simulink model "filtros_fir"  (R2014a)
settings: Solver=ode45  StartTime=0.0  StopTime=10.0  RelTol=1e-3
libraries: MCHP_Blockset x2
settings Model: Creator=Wels  LastModifiedBy=Wels

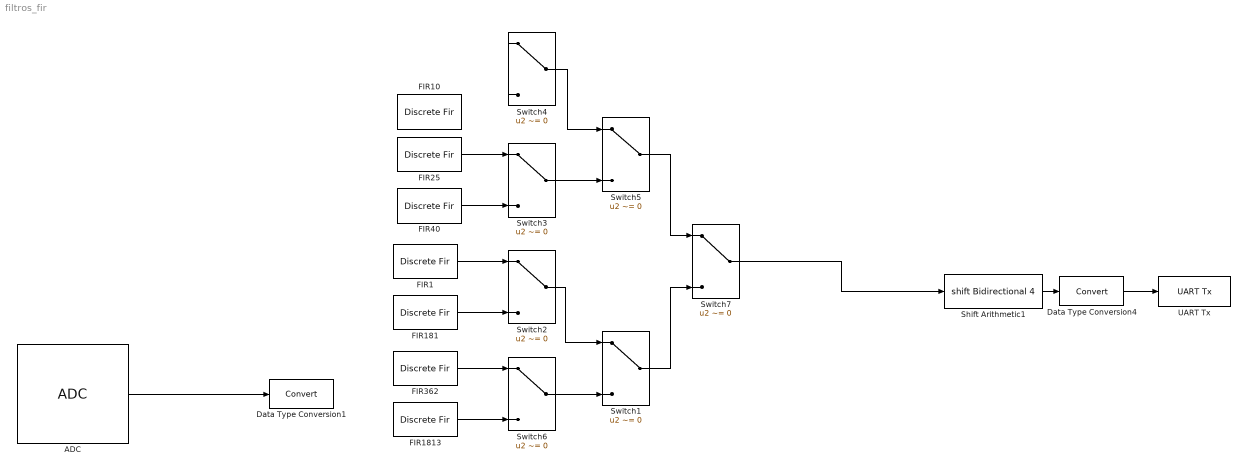
== system filtros_fir ==
  ADC : MCHP_Blockset/Analog IO/ADC  Priority=5  ADC_REF=1  Mode=12 bits  FORM=0000 dddd dddd dddd ==> Unsigned integer  ADC_R="< 5    kOhm"  nSAMPLECHANNELS=CH0 only  nSAMPLECHANNELS_12bits=CH0 only  SIMULTANEOUS=Simultaneously on all Channels  ADxCSS=[0]  MUXA_CH0N=off  MUXA_CH123=Dynamic Options  MUXA_CH123_TXT=AN0 : AN1 : AN2  MUXB_CH0=AN1  MUXB_CH0N=on  MUXB_CH123=Dynamic Options  MUXB_CH123_TXT=AN0 : AN1 : AN2  SequenceRepeat=1  SequenceTiming=are done as fast as possible at end of previous time step  SSRC_SSRCG=Dynamic Options  SSRC_SSRCG_TXT=0  Update_BlockOutput=After all trig and conversion sequence  Trig_TimeStep=with each update of the ADC block output  ADC_DMA_CHANNEL=use DMA Channel 0  SampleTime=0.001  Info=Total Time for Sample & Conversion : 9.45e-06s including 0s (x 1) sample time.  MCHP_PORT={Analog Input 0}{AN0}15:2:A0;  MCHP_MASTERLINK=ADC_DSPIC33/Microchip Master  ADC_TIMING=[9.4499999999999993e-06]
  Data Type Conversion1 : DataTypeConversion
  Data Type Conversion4 : DataTypeConversion
  FIR1 : DiscreteFir  Tag=BlockMethodSubSystem  Coefficients=[-2.9323800933922057e-18 -0.0015228449366636073 -0.003018760535505417 -0.0043911540093978458 -0.0055466659235829602 -0.006401109439598384 -0.0068851121818910791 -0.0069491080760650491 -0.0065673515956200142 -0.0057406721770929675 -0.0044977500977790479 -0.002894773705028665 -0.0010134274197902613 0.0010427444668100105 0.0031534568919988934 0.0051880532674748276 0.0070128109723885373 0.0084988032998812423 0.0095298916645369987 0.010010398197200024 0.0098720098997901601 0.009079491954896806 0.0076348388043248989 0.0055795650340087688 0.0029949304160725048 -3.0714546289964412e-18 -0.003252444656358322 -0.0065820093502685917 -0.0097885587309644792 -0.012661504624490524 -0.014990073316292731 -0.016574048280221781 -0.017234444684547753 -0.016823560059853641 -0.015233863006149173 -0.012405228378154698 -0.0083301010511404264 -0.0030562676555698828 0.0033129682426820939 0.010621283060200347 0.01866444257636788 0.027197829873822289 0.035946071730047706 0.0446143319962145 0.052900750057141198 0.060509437929656872 0.06716341457002048 0.072616852612101865 0.076666041454452896 0.079158530052541462 0.080000000000000002 0.079158530052541462 0.076666041454452896 0.072616852612101865 0.06716341457002048 0.060509437929656872 0.052900750057141198 0.0446143319962145 0.035946071730047706 0.027197829873822289 0.01866444257636788 0.010621283060200347 0.0033129682426820939 -0.0030562676555698828 -0.0083301010511404264 -0.012405228378154698 -0.015233863006149173 -0.016823560059853641 -0.017234444684547753 -0.016574048280221781 -0.014990073316292731 -0.012661504624490524 -0.0097885587309644792 -0.0065820093502685917 -0.003252444656358322 -3.0714546289964412e-18 0.0029949304160725048 0.0055795650340087688 0.0076348388043248989 0.009079491954896806 0.0098720098997901601 0.010010398197200024 0.0095298916645369987 0.0084988032998812423 0.0070128109723885373 0.0051880532674748276 0.0031534568919988934 0.0010427444668100105 -0.0010134274197902613 -0.002894773705028665 -0.0044977500977790479 -0.0057406721770929675 -0.0065673515956200142 -0.0069491080760650491 -0.0068851121818910791 -0.006401109439598384 -0.0055466659235829602 -0.0043911540093978458 -0.003018760535505417 -0.0015228449366636073 -2.9323800933922057e-18]  InputProcessing=Columns as channels (frame based)
  FIR10 : DiscreteFir  Tag=BlockMethodSubSystem  Coefficients=[0.05693190881682296 0.064608222044922184 0.071056300974898803 0.075931585257515435 0.078968604608715479 0.080000000000000002 0.078968604608715479 0.075931585257515435 0.071056300974898803 0.064608222044922184 0.05693190881682296]  InputProcessing=Columns as channels (frame based)
  FIR181 : DiscreteFir  Tag=BlockMethodSubSystem  Coefficients=[-0.0022639883275030691 -0.0016133097538512582 -0.00084337344267178184 2.9443416248695584e-18 0.00086517641377111313 0.0016978131053387859 0.0024442123003697996 0.0030547195836404385 0.0034869560845998604 0.003708678283102423 0.0037000773326903952 0.0034553599178999222 0.0029834933057486866 0.0023080461643020054 0.0014661110869005709 0.00050635136262791396 -0.00051373005733820136 -0.0015311506685924538 -0.0024812459539193805 -0.0033016804917040386 -0.0039364294880122191 -0.0043394827542988946 -0.0044780334288872089 -0.0043349388843936772 -0.0039102801218845766 -0.0032218965099678034 -0.0023048322069548306 -0.0012096956199982533 3.0290297657205514e-18 0.0012513822618214151 0.0024664608508178859 0.0035668251972659718 0.0044785243876568756 0.0051368355744426308 0.0054906248202151566 0.0055060198236647657 0.0051691468796323733 0.0044877332357838159 0.0034914382478542848 0.00223084906371908 0.0007751549565775495 -0.00079140561269844506 -0.0023741542968877447 -0.0038733985661101879 -0.005190376874854942 -0.0062333851575417194 -0.0069237239799580944 -0.0072011036523168346 -0.0070281638123607104 -0.0063938039032713691 -0.0053150798729646688 -0.0038374974349784778 -0.0020336194772699002 3.0861621459651029e-18 0.0021474459298498633 0.0042794328011263498 0.0062603671781829252 0.0079561219027827548 0.0092421084067647388 0.010011201898530072 0.010181066581124654 0.0097004455811658952 0.0085540225930631104 0.00676552764947183 0.0043988448641004351 0.0015569812197178019 -0.0016211327142456927 -0.0049659227570060362 -0.0082843295155859021 -0.011368535968756527 -0.01400586195480538 -0.015989349523563991 -0.017128513034918618 -0.017259704669759533 -0.016255551437491036 -0.014032954062411557 -0.010559199993407797 -0.0058558293809127396 3.1149317064883305e-18 0.0068767805961167097 0.014592556181376771 0.022921323366296955 0.031601672190584421 0.040347287698284315 0.048858835554886501 0.05683667922089531 0.063993828108091844 0.070068498248876995 0.074835680459695922 0.078117155278273911 0.079789466969549874 0.079789466969549874 0.078117155278273911 0.074835680459695922 0.070068498248876995 0.063993828108091844 0.05683667922089531 0.048858835554886501 0.040347287698284315 0.031601672190584421 0.022921323366296955 0.014592556181376771 0.0068767805961167097 3.1149317064883305e-18 -0.0058558293809127396 -0.010559199993407797 -0.014032954062411557 -0.016255551437491036 -0.017259704669759533 -0.017128513034918618 -0.015989349523563991 -0.01400586195480538 -0.011368535968756527 -0.0082843295155859021 -0.0049659227570060362 -0.0016211327142456927 0.0015569812197178019 0.0043988448641004351 0.00676552764947183 0.0085540225930631104 0.0097004455811658952 0.010181066581124654 0.010011201898530072 0.0092421084067647388 0.0079561219027827548 0.0062603671781829252 0.0042794328011263498 0.0021474459298498633 3.0861621459651029e-18 -0.0020336194772699002 -0.0038374974349784778 -0.0053150798729646688 -0.0063938039032713691 -0.0070281638123607104 -0.0072011036523168346 -0.0069237239799580944 -0.0062333851575417194 -0.005190376874854942 -0.0038733985661101879 -0.0023741542968877447 -0.00079140561269844506 0.0007751549565775495 0.00223084906371908 0.0034914382478542848 0.0044877332357838159 0.0051691468796323733 0.0055060198236647657 0.0054906248202151566 0.0051368355744426308 0.0044785243876568756 0.0035668251972659718 0.0024664608508178859 0.0012513822618214151 3.0290297657205514e-18 -0.0012096956199982533 -0.0023048322069548306 -0.0032218965099678034 -0.0039102801218845766 -0.0043349388843936772 -0.0044780334288872089 -0.0043394827542988946 -0.0039364294880122191 -0.0033016804917040386 -0.0024812459539193805 -0.0015311506685924538 -0.00051373005733820136 0.00050635136262791396 0.0014661110869005709 0.0023080461643020054 0.0029834933057486866 0.0034553599178999222 0.0037000773326903952 0.003708678283102423 0.0034869560845998604 0.0030547195836404385 0.0024442123003697996 0.0016978131053387859 0.00086517641377111313 2.9443416248695584e-18 -0.00084337344267178184 -0.0016133097538512582 -0.0022639883275030691]  InputProcessing=Columns as channels (frame based)
  FIR1813 : DiscreteFir  Tag=BlockMethodSubSystem  Coefficients=[0.00032952911187119737 0.00032473517058408992 0.00029949947214209755 0.00025535873427201875 0.00019504278155501242 0.00012230579388882381 4.1692698517550693e-05 -4.1744761582324127e-05 -0.00012276454860099542 -0.00019626361161977597 -0.00025759924854245692 -0.00030288231409216285 -0.00032922376001048669 -0.00033491888265804487 -0.00031955753227915043 -0.00028405316575898459 -0.00023058871159179856 -0.00016248244320140519 -8.3982096279824835e-05 -6.6378809126254589e-19 8.4194265639719084e-05 0.00016330446084229693 0.00023234078908090157 0.00028693456551297903 0.00032361461065292786 0.00034002788653010461 0.00033509035547182875 0.00030905839515836395 0.00026351607613477046 0.00020127888834994712 0.00012621976019108465 4.3028116193721218e-05 -4.3083041127590029e-05 -0.00012670373238769583 -0.00020256682711292391 -0.00026587975187858034 -0.0003126271945743762 -0.00033982568954094315 -0.00034571394614225253 -0.00032986678380497633 -0.00029322531066992586 -0.00023804123246993393 -0.0001677385741200386 -8.6701299773445198e-05 1.7095769056652346e-18 8.6925318595543704e-05 0.00016860650087831315 0.00023989116296424423 0.00029626763732437309 0.00033415045389244166 0.00035110829718730557 0.00034601995103387403 0.00031914823459720516 0.0002721270659772768 0.00020786224138893871 0.00013035194690182514 4.4438084316086506e-05 -4.4496126492876797e-05 -0.00013086338682871302 -0.0002092232772418191 -0.00027462489353193199 -0.00032291958567181065 -0.00035102404877583029 -0.00035711708646546684 -0.00034075749539601774 -0.00030291544841017098 -0.0002459151748724359 -0.0001732923105356631 -8.9574665622856739e-05 4.2406091449575885e-18 8.9811607478043859e-05 0.00017421030583805502 0.00024787182406707563 0.00030613328248453022 0.00034528828751800633 0.0003628226390728592 0.00035757566579229744 0.00032981684192100972 0.00028123264099433977 0.00021482421448547933 0.00013472209444100291 4.5929355051342866e-05 -4.5990801287047665e-05 -0.0001352635294002786 -0.00021626507313371292 -0.00028387696388909773 -0.00033380938205546812 -0.00036287325745926619 -0.00036918385463395836 -0.00035228285218252104 -0.00031317101754854693 -0.00025424918107297564 -0.00017917097527751953 -9.2616364891862638e-05 6.9431773108757513e-18 9.2867437590043943e-05 0.00018014371864827212 0.00025632252324914645 0.00031658076277386844 0.00035708386391707981 0.00037522969629670582 0.00036981563229449645 0.00034111802080524176 0.0002908788368540374 0.00022220009372350599 0.00013935240789474931 4.7509524650286494e-05 -4.7574698191683825e-05 -0.0001399266862029288 -0.00022372835517093937 -0.00029368356651569014 -0.00034535275480525611 -0.00037543458956305632 -0.0003819768071617564 -0.0003645027548861563 -0.00032404545418710423 -0.00026308678495157249 -0.00018540535425814439 -9.5842367054886074e-05 -1.1357237884133027e-18 9.6108934286664861e-05 0.00018643812916845751 0.00026528808170405533 0.00032766563145260981 0.00036960006498509737 0.00038839577976460714 0.00038280543597178358 0.00035311248165536272 0.00030111760635609418 0.00023002970645582749 0.00014426795378438256 4.9187169506072944e-05 -4.9256436000125337e-05 -0.00014487829737313407 -0.00023165394499001139 -0.00030409847902950876 -0.00035761316967114259 -0.00038877728673591022 -0.00039556664557550373 -0.0003774849135906076 -0.00033559917005555645 -0.00027247721077334916 -0.00019203026271991702 -9.9270734439122545e-05 1.5660508920444814e-18 9.9554341743169492e-05 0.00019312905719755106 0.00027481922546352311 0.00033945077011317867 0.00038290807863803977 0.0004023959708928867 0.00039661934827089863 0.0003658689858877898 0.00031200780106085897 0.00023835817568389076 0.000149497136030437 5.0972009405889051e-05 -5.1045784082619642e-05 -0.00015014720373929166 -0.00024008812831618706 -0.0003151826869550116 -0.00037066261021507856 -0.00040297989608681161 -0.00041003358581188909 -0.00039130616247513871 -0.00034790072846635657 -0.00028247633377206216 -0.00019908522633863289 -0.00010292197647182632 4.4671457703022416e-18 ...(+37954 chars)]  InputProcessing=Columns as channels (frame based)
  FIR25 : DiscreteFir  Tag=BlockMethodSubSystem  Coefficients=[2.9323800933922057e-18 0.0065349003912518319 0.013986521520040542 0.022140617857123224 0.030738535363382793 0.03948803959916064 0.048076271039389107 0.056184162411385824 0.063501554247964775 0.069742190535843199 0.074657770305471507 0.078050274193107061 0.079781875233049623 0.079781875233049623 0.078050274193107061 0.074657770305471507 0.069742190535843199 0.063501554247964775 0.056184162411385824 0.048076271039389107 0.03948803959916064 0.030738535363382793 0.022140617857123224 0.013986521520040542 0.0065349003912518319 2.9323800933922057e-18]  InputProcessing=Columns as channels (frame based)
  FIR362 : DiscreteFir  Tag=BlockMethodSubSystem  Coefficients=[0.001650376463598012 0.0015825312381259821 0.0014137541142797785 0.0011534389876633536 0.00081687731511497137 0.00042436792057086193 -2.9443416248695584e-18 -0.00042981815723557644 -0.00083799530578435738 -0.0011984573172655253 -0.0014878049656743924 -0.0016868245110408654 -0.0017817540857271033 -0.0017652230022217048 -0.0016368006040616255 -0.0014031150168812734 -0.0010775286887804811 -0.00067938530882542033 -0.00023286983616308538 0.00023445175067010767 0.00069332535466836039 0.0011146308883434818 0.0014712206979457768 0.0017396588106842526 0.0019017502063388319 0.0019457610091587563 0.0018672485707222357 0.0016694438216902552 0.001363155614300217 0.00096619639690671139 0.00050235863089377164 -2.9900643926682362e-18 -0.00050967914239235927 -0.00099456212774707274 -0.0014236278880093371 -0.0017689231276923855 -0.0020073701439448552 -0.00212229420857772 -0.0021045703518973967 -0.0019533118255606291 -0.0016760501587016992 -0.0012883879025936647 -0.00081313798312260797 -0.0002789960163697435 0.00028117804546945387 0.00083236689686450103 0.0013395697848544248 0.0017700092969748626 0.0020952328651794904 0.002292975287114482 0.0023486614765650684 0.0022564493297148377 0.0020197398593347592 0.0016511140022351931 0.0011716908076213678 0.00060993790674949478 -3.0290297657205514e-18 -0.00062035762153668083 -0.0012120677869352822 -0.0017372011997381944 -0.002161376119638383 -0.0024559862151476547 -0.0026001036683030768 -0.0025819325314929858 -0.0023997133688734491 -0.0020620128714468264 -0.0015873694898125741 -0.0010033059318942542 -0.0003447591850018573 0.00034798393840984587 0.0010317252326933607 0.0016630214593934425 0.002200915696405677 0.0026095637091342822 0.002860588824081117 0.0029350126780976166 0.0028246328773248067 0.0025327507330231672 0.0020741910030118225 0.0014745986694388476 0.00076904262821737293 -3.0611001307298754e-18 -0.00078516514306091923 -0.0015370810642747115 -0.0022074328391167796 -0.0027520241953703081 -0.0031336452659706947 -0.0033245630019182832 -0.0033084707358693767 -0.0030817636797847775 -0.0026540463164303561 -0.0020478234584631765 -0.0012973765011932551 -0.00044687709116363657 0.00045216103951341069 0.0013439480039284118 0.0021718220572704817 0.0028817878659493463 0.0034259714532140916 0.0037657747682680659 0.0038745264796302224 0.003739452107792216 0.0033628246369228321 0.0027622041970060533 0.0019697295818268345 0.0010304820912716735 -3.0861621459651029e-18 -0.0010589236803066702 -0.0020799799670867931 -0.0029974014299761721 -0.0037500955504258414 -0.0042856001195180427 -0.0045636112690340637 -0.0045588544915404153 -0.0042631032996302805 -0.0036861972694254464 -0.0028559685615458701 -0.0018170503878126201 -0.000628608568321545 0.00063889571099136724 0.0019077416398559281 0.0030975591825325474 0.0041302488474143587 0.0049349189973320797 0.0054525392096707202 0.00564001643742508 0.0054734268443363014 0.0049501791008919639 0.0040899425197108838 0.0029342426418104976 0.0015447039577525786 -3.1041271889287381e-18 -0.0016083495985849943 -0.0031811220401705377 -0.0046171982102015691 -0.0058197087123549891 -0.0067021633651109698 -0.0071941973827430242 -0.0072465775548062666 -0.0068351429706062661 -0.0059634059808752367 -0.0046636077383145347 -0.0029961053330960444 -0.0010470598678813219 0.0010755082322271531 0.0032471342243677796 0.0053335420608483378 0.0071981648230940347 0.0087101600273670355 0.0097524855407006093 0.010229583261543874 0.010074223906405224 0.0092530974901423747 0.0077707892859406862 0.005671857732794377 0.00304082520616346 -3.1149317064883305e-18 -0.0032948373128426009 -0.0066607338881747545 -0.009895590686091478 -0.012787554460655836 -0.015125332500993696 -0.016708925633011816 -0.017360239081873521 -0.016933022725857744 -0.015321612993337369 -0.012467997575705108 -0.0083667991296579435 -0.0030678716680886124 0.0033236814222058183 0.010650131669098508 0.018706323554951498 0.027247246796400379 0.035997660812390378 0.04466334170949824 0.052943435189128703 0.06054333727750718 ...(+4170 chars)]  InputProcessing=Columns as channels (frame based)
  FIR40 : DiscreteFir  Tag=BlockMethodSubSystem  Coefficients=[-0.01423297720420574 -0.015817959399409564 -0.016528271678139684 -0.016208243927688132 -0.014739975184467713 -0.012051521623166995 -0.0081230763316393183 -0.0029907383172590989 0.0032524116635554981 0.010458071899141172 0.01842731038110863 0.026917825484855638 0.03565356953724233 0.044336295104620511 0.05265847282390991 0.060316947197958951 0.067026647996413058 0.072533662871220136 0.076627002551852536 0.079148452405864642 0.080000000000000002 0.079148452405864642 0.076627002551852536 0.072533662871220136 0.067026647996413058 0.060316947197958951 0.05265847282390991 0.044336295104620511 0.03565356953724233 0.026917825484855638 0.01842731038110863 0.010458071899141172 0.0032524116635554981 -0.0029907383172590989 -0.0081230763316393183 -0.012051521623166995 -0.014739975184467713 -0.016208243927688132 -0.016528271678139684 -0.015817959399409564 -0.01423297720420574]  InputProcessing=Columns as channels (frame based)
  Shift Arithmetic1 : ArithShift  BitShiftNumber=4
  Switch{1..7} (7 alike) : Switch  Criteria=u2 ~= 0
  UART Tx : MCHP_Blockset/BUS UART/UART Tx  UART_REF=1  ORDERING=None  AllOrNothing=off  SampleTime=-1  MCHP_MASTERLINK=ADC_DSPIC33/Microchip Master  NSend_Input=off  UART_String=off  NSend_Output=off
  wires:
  Shift Arithmetic1/1 -> Data Type Conversion4/1
  Data Type Conversion4/1 -> UART Tx/1
  ADC/1 -> Data Type Conversion1/1
  ? -> Switch3/2, Switch2/2, Switch6/2
  ? -> Switch5/2, Switch1/2
  ? -> Switch7/2
  FIR362/1 -> Switch6/1
  Switch6/1 -> Switch1/3
  Switch2/1 -> Switch1/1
  FIR181/1 -> Switch2/3
  Switch4/1 -> Switch5/1
  Switch3/1 -> Switch5/3
  Switch5/1 -> Switch7/1
  Switch1/1 -> Switch7/3
  Switch7/1 -> Shift Arithmetic1/1
  ? -> FIR362/1
  ? -> FIR181/1
  ? -> FIR1/1
  ? -> FIR40/1
  ? -> FIR25/1
  ? -> FIR1813/1
  FIR40/1 -> Switch3/3
  FIR25/1 -> Switch3/1
  FIR1/1 -> Switch2/1
  FIR1813/1 -> Switch6/3
